simulink model "controller_disc"  (R2023b)
settings: Solver=FixedStepAuto  StartTime=0.0  StopTime=1  RelTol=1e-3  EnableMultiTasking=on
undefined symbols (not defined in the file): C, F, G, k_awp, K_i_disc, K_r_disc, ke, L_disc, p, T, targetPos, tPWM, Vmax
libraries: simulink x2
settings Model: ExtModeTrigDuration=10  Creator=miqui  LastModifiedBy=miqui
settings OptimizationCC: EnhancedBackFolding=on  PassReuseOutputArgsAs=Individual arguments  ZeroExternalMemoryAtStartup=off  ZeroInternalMemoryAtStartup=off  MaxStackSize=64  OptimizeBlockOrder=speed  DifferentSizesBufferReuse=on  OptimizationCustomize=off  EfficientTunableParamExpr=on
settings DebuggingCC: ParameterTunabilityLossMsg=error
settings HardwareCC: ProdBitPerPointer=32  ProdBitPerSizeT=32  ProdBitPerPtrDiffT=32  ProdLargestAtomicInteger=Long  ProdLargestAtomicFloat=Double  ProdWordSize=32  ProdLongLongMode=on  ProdHWDeviceType=ARM Compatible->ARM Cortex  UseEmbeddedCoderFeatures=off
settings SFSimCC: MATLABDynamicMemAlloc=off
settings RTWCC: Description=Embedded Coder  SystemTargetFile=ert.tlc  HardwareBoard=STM32 Nucleo F411RE  TemplateMakefile=ert_default_tmf  Toolchain=GNU Tools for ARM Embedded Processors
settings CodeAppCC: ForceParamTrailComments=on  IgnoreCustomStorageClasses=off  OperatorAnnotations=on  SimulinkDataObjDesc=on  SFDataObjDesc=on  InsertBlockDesc=on
settings ERTTargetCC: SupportNonInlinedSFcns=on  ExtModeTransport=3  ExtModeStaticAlloc=on  ExtModeStaticAllocSize=2000  ExtModeMexFile=ext_xcp  ExtModeIntrfLevel=Level2 - Open

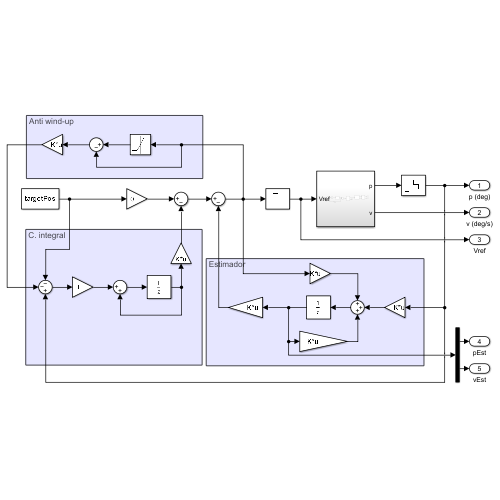
[thumbnail: Simulink's stored preview of the top-level diagram]
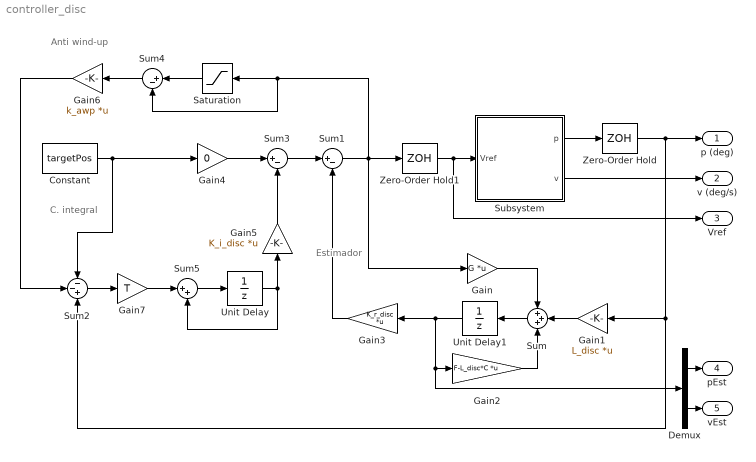
== system controller_disc ==
  note: Anti wind-up
  note: Estimador
  note: C. integral
  Constant : Constant  Value=targetPos
  Demux : Demux  Outputs=2
  Gain : Gain  Gain=G  Multiplication=Matrix(K*u)
  Gain1 : Gain  Gain=L_disc  Multiplication=Matrix(K*u)
  Gain2 : Gain  Gain=F-L_disc*C  Multiplication=Matrix(K*u)
  Gain3 : Gain  Gain=K_r_disc  Multiplication=Matrix(K*u)
  Gain4 : Gain  Gain=0
  Gain5 : Gain  Gain=K_i_disc  Multiplication=Matrix(K*u)
  Gain6 : Gain  Gain=k_awp  Multiplication=Matrix(K*u)
  Gain7 : Gain  Gain=T
  Saturation : Saturate  UpperLimit=12  LowerLimit=-12
  Subsystem : Subsystem
  Sum : Sum  Inputs=+++
  Sum1 : Sum  Inputs=|+-
  Sum2 : Sum  Inputs=--+
  Sum3 : Sum  Inputs=|+-
  Sum4 : Sum  Inputs=|+-
  Sum5 : Sum  Inputs=|++
  Unit Delay : UnitDelay  SampleTime=T  HasFrameUpgradeWarning=on
  Unit Delay1 : UnitDelay  SampleTime=T  HasFrameUpgradeWarning=on
  Zero-Order Hold : ZeroOrderHold  SampleTime=T
  Zero-Order Hold1 : ZeroOrderHold  SampleTime=T
  p (deg) : Outport
  v (deg/s) : Outport  Port=2
  Vref : Outport  Port=3
  pEst : Outport  Port=4
  vEst : Outport  Port=5
  wires:
  Sum/1 -> Unit Delay1/1
  Gain/1 -> Sum/1
  Gain1/1 -> Sum/2
  Gain2/1 -> Sum/3
  Unit Delay1/1 -> Demux/1, Gain2/1, Gain3/1
  Gain3/1 -> Sum1/2
  Sum1/1 -> Saturation/1, Sum4/2, Zero-Order Hold1/1, Gain/1
  Constant/1 -> Gain4/1, Sum2/1
  Subsystem/1(p) -> Zero-Order Hold/1
  Subsystem/2(v) -> v (deg/s)/1
  Zero-Order Hold/1 -> p (deg)/1, Sum2/3, Gain1/1
  Zero-Order Hold1/1 -> Vref/1, Subsystem/1(Vref)
  Gain4/1 -> Sum3/1
  Sum3/1 -> Sum1/1
  Saturation/1 -> Sum4/1
  Sum4/1 -> Gain6/1
  Gain5/1 -> Sum3/2
  Sum2/1 -> Gain7/1
  Gain7/1 -> Sum5/1
  Sum5/1 -> Unit Delay/1
  Unit Delay/1 -> Sum5/2, Gain5/1
  Gain6/1 -> Sum2/2
  Demux/2 -> vEst/1
  Demux/1 -> pEst/1

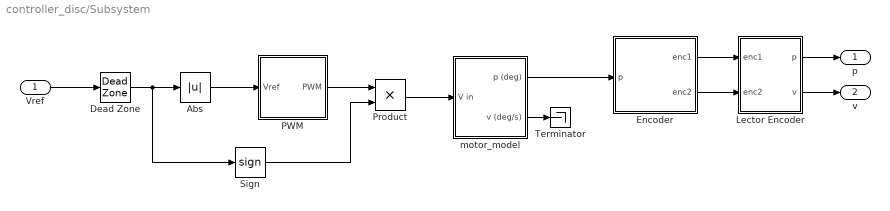
== system controller_disc/Subsystem ==
  Vref : Inport
  Abs : Abs  SaturateOnIntegerOverflow=off
  Dead Zone : DeadZone
  Encoder : Subsystem
  Lector Encoder : Subsystem
  PWM : Subsystem
  Product : Product
  Sign : Signum
  Terminator : Terminator
  motor_model : Subsystem
  p : Outport
  v : Outport  Port=2
  wires:
  Vref/1 -> Dead Zone/1
  Lector Encoder/1(p) -> p/1
  Lector Encoder/2(v) -> v/1
  Abs/1 -> PWM/1(Vref)
  Dead Zone/1 -> Sign/1, Abs/1
  Product/1 -> motor_model/1(V in)
  Sign/1 -> Product/2
  motor_model/1(p (deg)) -> Encoder/1(p)
  Encoder/1("enc1 ") -> Lector Encoder/1(enc1)
  Encoder/2("enc2 ") -> Lector Encoder/2(enc2)
  PWM/1(PWM) -> Product/1
  motor_model/2(v (deg/s)) -> Terminator/1

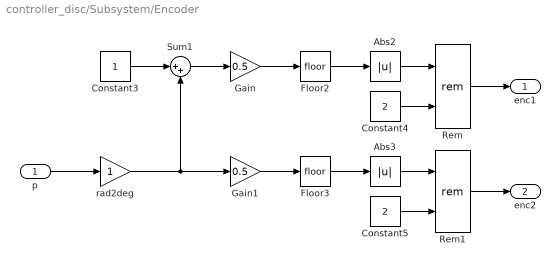
== system controller_disc/Subsystem/Encoder ==
  p : Inport
  Abs2 : Abs  SaturateOnIntegerOverflow=off
  Abs3 : Abs  SaturateOnIntegerOverflow=off
  Constant3 : Constant
  Constant4 : Constant  Value=2
  Constant5 : Constant  Value=2
  Floor2 : Rounding
  Floor3 : Rounding
  Gain : Gain  Gain=0.5
  Gain1 : Gain  Gain=0.5
  Rem : Math  Operator=rem
  Rem1 : Math  Operator=rem
  Sum1 : Sum  Inputs=|++
  rad2deg : Gain
  "enc1 " : Outport  SampleTime=0.0001
  "enc2 " : Outport  Port=2  SampleTime=0.0001
  wires:
  Constant4/1 -> Rem/2
  Constant3/1 -> Sum1/1
  p/1 -> rad2deg/1
  Rem1/1 -> "enc2 "/1
  Gain/1 -> Floor2/1
  Abs3/1 -> Rem1/1
  rad2deg/1 -> Gain1/1, Sum1/2
  Sum1/1 -> Gain/1
  Gain1/1 -> Floor3/1
  Floor3/1 -> Abs3/1
  Floor2/1 -> Abs2/1
  Constant5/1 -> Rem1/2
  Rem/1 -> "enc1 "/1
  Abs2/1 -> Rem/1

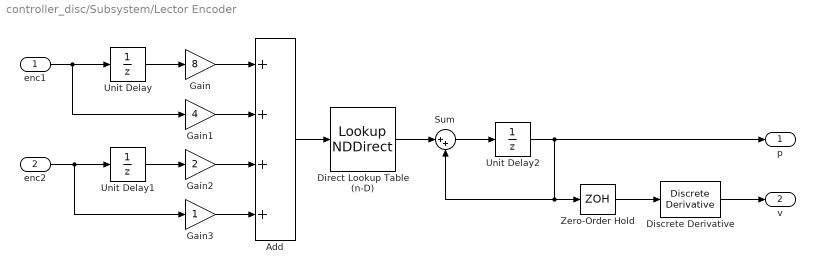
== system controller_disc/Subsystem/Lector Encoder ==
  enc1 : Inport
  enc2 : Inport  Port=2
  Add : Sum  Inputs=++++  OutDataTypeStr=double
  Direct Lookup Table (n-D) : LookupNDDirect  NumberOfTableDimensions=1  Table=[0,-1,1,0,1,0,0,-1,-1,0,0,1,0,1,-1,0]
  Discrete Derivative : simulink/Discrete/Discrete Derivative  gainval=1.0  ICPrevScaledInput=0.0  OutMin=[]  OutMax=[]  OutDataType=fixdt(1, 16)  OutScaling=2^-10  DoSatur=off
  Gain : Gain  Gain=8
  Gain1 : Gain  Gain=4
  Gain2 : Gain  Gain=2
  Gain3 : Gain
  Sum : Sum  Inputs=|++
  Unit Delay : UnitDelay  SampleTime=-1  HasFrameUpgradeWarning=on
  Unit Delay1 : UnitDelay  SampleTime=-1  HasFrameUpgradeWarning=on
  Unit Delay2 : UnitDelay  SampleTime=-1  HasFrameUpgradeWarning=on
  Zero-Order Hold : ZeroOrderHold  SampleTime=0.01
  p : Outport
  v : Outport  Port=2
  wires:
  enc1/1 -> Unit Delay/1, Gain1/1
  enc2/1 -> Unit Delay1/1, Gain3/1
  Unit Delay/1 -> Gain/1
  Unit Delay1/1 -> Gain2/1
  Gain/1 -> Add/1
  Gain1/1 -> Add/2
  Gain2/1 -> Add/3
  Gain3/1 -> Add/4
  Add/1 -> Direct Lookup Table (n-D)/1
  Direct Lookup Table (n-D)/1 -> Sum/1
  Sum/1 -> Unit Delay2/1
  Unit Delay2/1 -> Zero-Order Hold/1, Sum/2, p/1
  Zero-Order Hold/1 -> Discrete Derivative/1
  Discrete Derivative/1 -> v/1

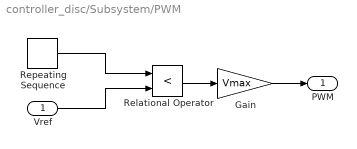
== system controller_disc/Subsystem/PWM ==
  Vref : Inport
  Gain : Gain  Gain=Vmax
  Relational Operator : RelationalOperator  Operator=<  OutDataTypeStr=boolean  RndMeth=Simplest  InputSameDT=off
  Repeating Sequence : simulink/Sources/Repeating Sequence  rep_seq_t=linspace(0,tPWM,100)  rep_seq_y=linspace(0,Vmax,100)
  PWM : Outport
  wires:
  Relational Operator/1 -> Gain/1
  Gain/1 -> PWM/1
  Vref/1 -> Relational Operator/2
  Repeating Sequence/1 -> Relational Operator/1

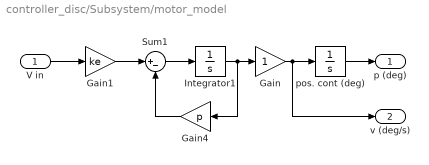
== system controller_disc/Subsystem/motor_model ==
  V in : Inport
  Gain : Gain
  Gain1 : Gain  Gain=ke
  Gain4 : Gain  Gain=p
  Integrator1 : Integrator
  Sum1 : Sum  Inputs=|+-
  pos. cont (deg) : Integrator
  p (deg) : Outport
  v (deg/s) : Outport  Port=2
  wires:
  Sum1/1 -> Integrator1/1
  Gain4/1 -> Sum1/2
  Integrator1/1 -> Gain/1, Gain4/1
  Gain1/1 -> Sum1/1
  Gain/1 -> pos. cont (deg)/1, v (deg/s)/1
  pos. cont (deg)/1 -> p (deg)/1
  V in/1 -> Gain1/1
